simulink model "Ej3_v3"  (R2015a)
settings: Solver=ode45  StartTime=0.0  StopTime=200  RelTol=1e-3
libraries: cstblocks x2, simulink x1
settings Model: Creator=Daniel  LastModifiedBy=Daniel

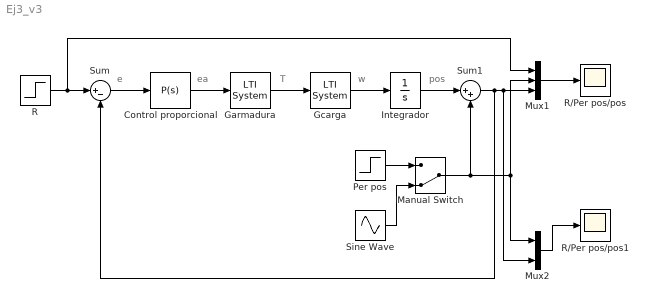
== system Ej3_v3 ==
  note: T
  note: pos
  note: w
  note: e
  note: ea
  Control proporcional : simulink/Continuous/PID Controller  Controller=P  TimeDomain=Continuous-time  SampleTime=-1  IntegratorMethod=Forward Euler  FilterMethod=Forward Euler  Form=Ideal  UseFilter=on  ControllerParametersSource=internal  P=1  I=0  D=0  N=100  InitialConditionSource=internal  InitialConditionForIntegrator=0  InitialConditionForFilter=0  ExternalReset=none  LimitOutput=off  UpperSaturationLimit=12  LowerSaturationLimit=-inf  LinearizeAsGain=on  AntiWindupMode=none  Kb=1  TrackingMode=off  Kt=1  PParamMin=[]  PParamMax=[]  IParamMin=[]  IParamMax=[]  DParamMin=[]  DParamMax=[]  NParamMin=[]  NParamMax=[]  KbParamMin=[]  KbParamMax=[]  KtParamMin=[]  KtParamMax=[]  POutMin=[]  POutMax=[]  IOutMin=[]  IOutMax=[]  DOutMin=[]  DOutMax=[]  NOutMin=[]  NOutMax=[]  KbOutMin=[]  KbOutMax=[]  KtOutMin=[]  KtOutMax=[]  IntegratorOutMin=[]  IntegratorOutMax=[]  FilterOutMin=[]  FilterOutMax=[]  SumOutMin=[]  SumOutMax=[]  SumI1OutMin=[]  SumI1OutMax=[]  SumI2OutMin=[]  SumI2OutMax=[]  SumI3OutMin=[]  SumI3OutMax=[]  SumDOutMin=[]  SumDOutMax=[]  SaturationOutMin=[]  SaturationOutMax=[]  IntegratorContinuousStateAttributes=''  IntegratorStateMustResolveToSignalObject=off  IntegratorRTWStateStorageClass=Auto  FilterContinuousStateAttributes=''  FilterStateMustResolveToSignalObject=off  FilterRTWStateStorageClass=Auto  DifferentiatorICPrevScaledInput=0  DifferentiatorOutMin=[]  DifferentiatorOutMax=[]
  Garmadura : cstblocks/LTI System  sys=Garm  IC=[]
  Gcarga : cstblocks/LTI System  sys=Gcar  IC=[]
  Integrador : Integrator
  Manual Switch : ManualSwitch  CurrentSetting=0
  Mux1 : Mux  Inputs=3
  Mux2 : Mux  Inputs=2
  Per pos : Step  Time=30  After=0.05  SampleTime=0
  R : Step  Time=0  After=0.6  SampleTime=0
  R/Per pos/pos : Scope
      settings: TimeRange=60  SaveName=pos
  R/Per pos/pos1 : Scope
      settings: TimeRange=60  SaveName=fre
  Sine Wave : Sin  Amplitude=0.05  Frequency=0.25  SampleTime=0  VectorParams1D=off
  Sum : Sum  Inputs=|+-
  Sum1 : Sum  Inputs=|++
  wires:
  Sum/1 -> Control proporcional/1
  Control proporcional/1 -> Garmadura/1
  Gcarga/1 -> Integrador/1
  Mux1/1 -> R/Per pos/pos/1
  R/1 -> Mux1/1, Sum/1
  Garmadura/1 -> Gcarga/1
  Manual Switch/1 -> Sum1/2, Mux2/1, Mux1/2
  Integrador/1 -> Sum1/1
  Sum1/1 -> Sum/2, Mux2/2, Mux1/3
  Sine Wave/1 -> Manual Switch/2
  Per pos/1 -> Manual Switch/1
  Mux2/1 -> R/Per pos/pos1/1
